simulink model "cop"  (R2020a)
settings: Solver=FixedStepAuto  StartTime=0.0  StopTime=300  FixedStep=1  RelTol=1e-3
undefined symbols (not defined in the file or in its folder): inf_depth, Kc_ini, PGravel
libraries: simulink x4
(part 1 of 2)
settings Model: Creator=KevinChan  LastModifiedBy=KevinChan

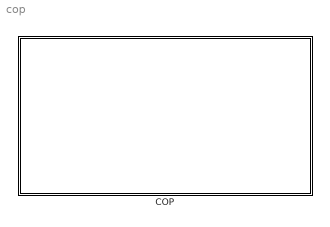
== system cop ==
  COP : Subsystem

== system cop/COP ==
  Climate Model : Subsystem
  Display : Display
  Economic Model : Subsystem
  Gain : Gain  Gain=0.001
  Gain1 : Gain  Gain=0.001
  Integrator : Integrator
  Optimal Irrigation Calculation : Subsystem
  Plant Model : Subsystem
  Scope : Scope  NumInputPorts=2
  Scope1 : Scope
  Soil Model : Subsystem
  Subtract : Sum  Inputs=++-
  VWC : Delay  DelayLength=1  InitialConditionSource=Input port  InitialCondition=0
      settings: InputPortMap=u0,p4
  initial vwc : Constant  Value=0.3
  tag scope: I=global, VWC=global
  wires:
  initial vwc/1 -> VWC/2
  Subtract/1 -> VWC/1, [VWC]
  VWC/1 -> Scope1/1, Subtract/1
  [I] -> Scope/1, Gain1/1
  [WL] -> Scope/2, Gain/1
  Gain/1 -> Subtract/3
  Gain1/1 -> Subtract/2
  Optimal Irrigation Calculation/1(Out1) -> Integrator/1, [I]
  Integrator/1 -> Display/1

== system cop/COP/Climate Model ==
  " Final Calculation for Data" : Subsystem
  " Historic Data" : Subsystem
  AI Forecast Prediction : Subsystem
  General Climate Database : Subsystem  mask{lcation=Palo Alto, Parameter7=No, LatDeg=37, LatMin=28, Altitude=9.1, WindH=2}
      mask prompts: lcation "Select Location"; Parameter7 "More specific Latitude?"; LatDeg "Latitude Degree"; LatMin "Latitude Minute"; Altitude "Altitude above Sea Level [m]"; WindH "Height of measurement above ground surface [m]"
      mask TypeOptions lcation: Palo Alto
      mask TypeOptions Parameter7: Yes | No
      mask DialogControl ParameterGroupVar Prompt: Location
      mask DialogControl Container4 Prompt: If yes, please fill out the following:
      mask DialogControl Container3 Prompt: Wind Measurement (Enter 2 if it uses COP AI Prediction)

== system cop/COP/Economic Model ==

== system cop/COP/Optimal Irrigation Calculation ==
  Constant : Constant  Value=0
  Constant1 : Constant  Value=0
  Display : Display
  Gain : Gain  Gain=0.001
  Gain1 : Gain  Gain=1000
  Math Function : Math  Operator=mod  SaturateOnIntegerOverflow=on
  MinMax : MinMax  Function=max  Inputs=2
  Subtract : Sum  Inputs=++-+
  Switch : Switch  Criteria=u2 ~= 0
  Water Runoff Adjustment : Constant  Value=0
  Out1 : Outport
  wires:
  [qFC] -> Display/1, Subtract/1
  [WL] -> Gain/1
  MinMax/1 -> Gain1/1
  Constant/1 -> MinMax/2
  [VWC] -> Subtract/3
  Subtract/1 -> MinMax/1
  Water Runoff Adjustment/1 -> Subtract/4
  Gain/1 -> Subtract/2
  [DafterPD] -> Math Function/1
  [interval_irr] -> Math Function/2
  Math Function/1 -> Switch/2
  Switch/1 -> Out1/1
  Gain1/1 -> Switch/3
  Constant1/1 -> Switch/1

== system cop/COP/Plant Model ==
  General Plant Database : Subsystem  mask{CropType=Maize (Sweet Corn), PD_Year=2021, PD_Month=2, PD_Day=28, interval_irr_choice=7 days, Parameter18=No, Lini=20, Ldev=40, Lmid=70, Llate=10, Kc_choice=Dual Crop Coefficient, Kc_mid=1.15, Kc_end=1.05, MaxCropH=1.5, Kcb_ini=0.15, Kcb_mid=1.10, Kcb_end=1.00, Zr=1.0}
      mask prompts: CropType "Crop Type"; PD_Year "Year"; PD_Month "Month"; PD_Day "Day"; interval_irr_choice "Interval of Irrigation (0 if unkwon)"; Parameter18 "More specific inputs?"; Lini "Initial Stage"; Ldev "Devloping Stage"; Lmid "Mid-season Stage"; Llate "Late Season Stage"; Kc_choice "Single or Dual Crop Coefficients"; Kc_mid "Enter Kc mid from the Table"; Kc_end "Enter Kc end from the Table"; MaxCropH "Enter Maximum Crop Height (h) (m) from the Table"; Kcb_ini "Enter Kcb ini from the Table"; Kcb_mid "Enter Kcb mid from the Table"; Kcb_end "Enter Kcb end from the Table"; Zr "Enter Zr from the Table"
      mask init:
      | interval_irr = 1;
      | if interval_irr_choice == 1
      |     interval_irr = 1;
      | elseif interval_irr_choice == 2
      |     interval_irr = 2;
      | elseif interval_irr_choice == 3
      |     interval_irr = 4;
      | elseif interval_irr_choice == 4
      |     interval_irr = 7;
      | elseif interval_irr_choice == 5
      |     interval_irr = 10;
      | elseif interval_irr_choice == 6
      |     interval_irr = 20;
      | end
      mask TypeOptions CropType: Maize (Sweet Corn)
      mask TypeOptions interval_irr_choice: 1 day | 2 days | 4 days | 7 days | 10 days | 20 days
      mask TypeOptions Parameter18: Yes | No
      mask TypeOptions Kc_choice: Single Crop Coefficient | Dual Crop Coefficient
      mask DialogControl ParameterGroupVar Prompt: General
      mask DialogControl Control2 Prompt: Plant Date:
      mask DialogControl Control12 Prompt: If yes, please fill out the following:
      mask DialogControl Container3 Prompt: Lengths of Crop Develop Stages
      mask DialogControl Control3 Prompt: Find the values in the following link with corresponding crop type and closest plant date:
      mask DialogControl Control4 Prompt: http://www.fao.org/3/x0490e/x0490e0b.htm#length%20of%20growth%20stages
      mask DialogControl Container4 Prompt: Single Crop Coefficients
      mask DialogControl Control5 Prompt: Find the values for your corresponding crop in the following table:
      mask DialogControl Control6 Prompt: http://www.fao.org/3/x0490e/x0490e0b.htm#tabulated%20kc%20values
      mask DialogControl Container5 Prompt: Dual Crop Coefficents
      mask DialogControl Control7 Prompt: Find the values for your corresponding crop in the following table:
      mask DialogControl Control8 Prompt: http://www.fao.org/3/x0490e/x0490e0c.htm#basal%20crop%20coefficient%20(kcb)
      mask DialogControl Container6 Prompt: Effective Rooting Depth
      mask DialogControl Control10 Prompt: Find the values for your corresponding crop in the following table:
      mask DialogControl Control9 Prompt: http://www.fao.org/3/x0490e/x0490e0e.htm#soil%20water%20availability
  Plant Data Calculation : Subsystem

== system cop/COP/Soil Model ==
  Add : Sum
  Constant : Constant
  Crop Evapotranspiration (ETc) [mm/day] : Product
  Display : Display
  Dual Crop Coefficient (Kcb + Ke) : Subsystem
  Evaporation (ETe) [mm/day] : Product
  General Soil Database : Subsystem  mask{PSand=0.489, PClay=0.170, PSilt=0.341, POM=0.05, fw_choice=Precipitation (fw = 1.0), fw_measured=1, SM_choice=Estimated Soil Moisture Value, qFC_measured=0, qWP_measured=0, Ze_choice=Estimated, Ze_measured=0}
      mask prompts: PSand "Percentage of Sand"; PClay "Percentage of Clay"; PSilt "Percentage of Silt"; POM "Percentage of Organic Matter (0.03-0.06 if unkown)"; fw_choice "Please select the following method (average fw of that method)"; fw_measured "If you selected others or specific fw, please enter your fw value"; SM_choice "Estimated or measured?"; qFC_measured "Field Capacity Soil Moisture (% Volume in m)"; qWP_measured "Wiliting Point Soil Moisture (% Volume in m)"; Ze_choice "Ze estimated or measured?"; Ze_measured "Enter Ze measured if selected"
      mask init:
      | fw = 1
      | if fw_choice == 5
      |     fw = 0.8
      | elseif fw_choice == 6
      |     fw = 0.5
      | elseif fw_choice == 7
      |     fw = 0.4
      | elseif fw_choice == 8
      |     fw = fw_measured
      | end
      mask TypeOptions fw_choice: Precipitation (fw = 1.0) | Sprinkler Irrigation (fw = 1.0) | Basin Irrigation (fw = 1.0) | Border Irrigation (fw = 1.0) | Furrow irrigation (every furrow), narrow bed (fw = 0.6 ... 1.0) | Furrow irrigation (every furrow), wide bed (fw = 0.4 ... 0.6) | Furrow irrigation (alternated furrows) (fw = 0.3 ... 0.5) | Trickle irrigation (fw = 0.3 ... 0.4) | Others or specific fw
      mask TypeOptions SM_choice: Estimated Soil Moisture Value | Measured Soil Moisture Value
      mask TypeOptions Ze_choice: Estimated | Measured
      mask DialogControl ParameterGroupVar Prompt: Percentage of Soil Content (add up to 1)
      mask DialogControl Container7 Prompt: Weight Percentage of Organic Matter
      mask DialogControl Container6 Prompt: Fraction of soil surface wetted by irrigation or precipitation
      mask DialogControl Container3 Prompt: Soil Moisture Data (more accurate if measured)
      mask DialogControl Control3 Prompt: Fill the following if you selected measured
      mask DialogControl Container8 Prompt: Ze depth of the surface soil layer that is subject to drying by way of evaporation [0.10-0.15m]
  Index Vector : MultiPortSwitch  Inputs=2
  Product : Product
  Reference Evapotraspiration (ET0) [mm/day] : Subsystem
  Scope1 : Scope
  Single Crop Coefficient (Kc) : Subsystem
  Soil Data Calculation : Subsystem
  tag scope: E=global, ET0=global, WL=global
  wires:
  Reference Evapotraspiration (ET0) [mm/day]/1(ET0) -> Evaporation (ETe) [mm/day]/1, Crop Evapotranspiration (ETc) [mm/day]/1, [ET0], Display/1
  Single Crop Coefficient (Kc)/1(Out1) -> Index Vector/2
  Index Vector/1 -> Crop Evapotranspiration (ETc) [mm/day]/2
  Dual Crop Coefficient (Kcb + Ke)/2(Ke) -> Evaporation (ETe) [mm/day]/2, Add/2
  Add/1 -> Index Vector/3
  Evaporation (ETe) [mm/day]/1 -> [E]
  [Kc_choice] -> Index Vector/1
  Dual Crop Coefficient (Kcb + Ke)/1(Kcb) -> Scope1/1, Add/1
  Product/1 -> [WL]
  Constant/1 -> Product/2
  Crop Evapotranspiration (ETc) [mm/day]/1 -> Product/1

== system cop/COP/Climate Model/ Final Calculation for Data ==
  Atmospheric Pressure [kPa] : Subsystem
  Daily Temperature [°C] : Subsystem
  Goto12 : Goto  Commented=on  GotoTag=Tpast  TagVisibility=global
  Goto13 : Goto  Commented=on  GotoTag=Tpast_t  TagVisibility=global
  Humidity : Subsystem
  Net Radiation at the Crop Surface (Rn) [MJ/m^2/day] : Subsystem
  Precipitation [mm/day] : Subsystem
  Wind Speed : Subsystem
  tag scope: AP=global, P=global, RHmax=global, RHmean=global, RHmin=global, Rn=global, Tdew=global, Tdry=global, Tmax=global, Tmean=global, Tmin=global, Twet=global, u2=global
  wires:
  Daily Temperature [°C]/1(Tmax) -> [Tmax]
  Daily Temperature [°C]/2(Tmin) -> [Tmin]
  Daily Temperature [°C]/3(Tmean) -> [Tmean]
  Net Radiation at the Crop Surface (Rn) [MJ/m^2/day]/1(Rn) -> [Rn]
  Wind Speed/1(Out1) -> [u2]
  Atmospheric Pressure [kPa]/1(P) -> [AP]
  Daily Temperature [°C]/4(Tdew) -> [Tdew]
  Daily Temperature [°C]/5(Tdry) -> [Tdry]
  Daily Temperature [°C]/6(Twet) -> [Twet]
  Humidity/1(RHmax) -> [RHmax]
  Humidity/3(RHmean) -> [RHmean]
  Humidity/2(RHmin) -> [RHmin]
  Daily Temperature [°C]/7(Tpast) -> Goto12/1
  Daily Temperature [°C]/8(Tpast_time) -> Goto13/1
  Precipitation [mm/day]/1(P) -> [P]

== system cop/COP/Climate Model/ Historic Data ==
  Humidity : Subsystem
  Precipitation : Subsystem
  Solar Radiation : Subsystem
  Temperature [°C] : Subsystem
  "Wind Speed " : Subsystem

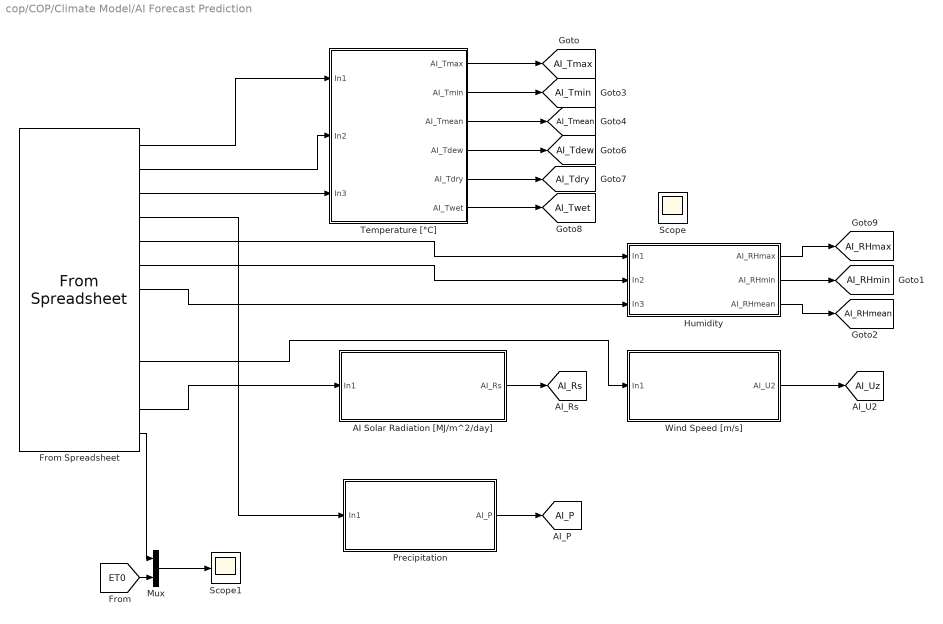
== system cop/COP/Climate Model/AI Forecast Prediction ==
  AI Solar Radiation [MJ/m^2/day] : Subsystem
  From Spreadsheet : FromSpreadsheet  FileName=paloalto3.2020.xlsx  Range=B11:N376  TreatFirstColumnAs=Data  SampleTime=[0,1]
  Humidity : Subsystem
  Mux : Mux  Inputs=2
  Precipitation : Subsystem
  Scope : Scope
  Scope1 : Scope
  Temperature [°C] : Subsystem
  Wind Speed [m/s] : Subsystem
  tag scope: AI_P=global, AI_RHmax=global, AI_RHmean=global, AI_RHmin=global, AI_Rs=global, AI_Tdew=global, AI_Tdry=global, AI_Tmax=global, AI_Tmean=global, AI_Tmin=global, AI_Twet=global, AI_Uz=global
  wires:
  AI Solar Radiation [MJ/m^2/day]/1(AI_Rs) -> [AI_Rs]
  Wind Speed [m/s]/1(AI_U2) -> [AI_Uz]
  Precipitation/1(AI_P) -> [AI_P]
  Humidity/1(AI_RHmax) -> [AI_RHmax]
  Humidity/2(AI_RHmin) -> [AI_RHmin]
  Humidity/3(AI_RHmean) -> [AI_RHmean]
  Temperature [°C]/1(AI_Tmax) -> [AI_Tmax]
  Temperature [°C]/2(AI_Tmin) -> [AI_Tmin]
  Temperature [°C]/3(AI_Tmean) -> [AI_Tmean]
  Temperature [°C]/4(AI_Tdew) -> [AI_Tdew]
  Temperature [°C]/5(AI_Tdry) -> [AI_Tdry]
  Temperature [°C]/6(AI_Twet) -> [AI_Twet]
  [ET0] -> Mux/2
  Mux/1 -> Scope1/1
  From Spreadsheet/1 -> Temperature [°C]/1(In1)
  From Spreadsheet/2 -> Temperature [°C]/2(In2)
  From Spreadsheet/3 -> Temperature [°C]/3(In3)
  From Spreadsheet/13 -> Mux/1
  From Spreadsheet/4 -> Precipitation/1(In1)
  From Spreadsheet/5 -> Humidity/1(In1)
  From Spreadsheet/6 -> Humidity/2(In2)
  From Spreadsheet/7 -> Humidity/3(In3)
  From Spreadsheet/10 -> Wind Speed [m/s]/1(In1)
  From Spreadsheet/12 -> AI Solar Radiation [MJ/m^2/day]/1(In1)

== system cop/COP/Climate Model/General Climate Database ==
  Altitude : Constant  Value=Altitude
  LatDeg : Constant  Value=LatDeg
  LatMin : Constant  Value=LatMin
  WindH : Constant  Value=WindH
  tag scope: Altitude=global, LatDeg=global, LatMin=global, WindH=global
  wires:
  Altitude/1 -> [Altitude]
  LatDeg/1 -> [LatDeg]
  LatMin/1 -> [LatMin]
  WindH/1 -> [WindH]

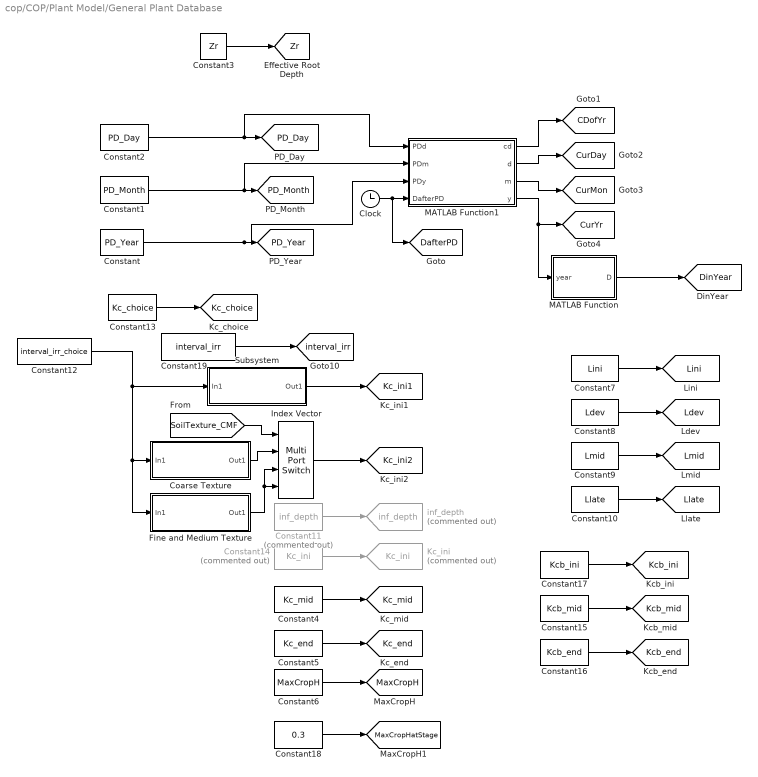
== system cop/COP/Plant Model/General Plant Database ==
  Clock : Clock
  Coarse Texture : Subsystem
  Constant : Constant  Value=PD_Year
  Constant1 : Constant  Value=PD_Month
  Constant10 : Constant  Value=Llate
  Constant11 : Constant  Commented=on  Value=inf_depth
  Constant12 : Constant  Value=interval_irr_choice
  Constant13 : Constant  Value=Kc_choice
  Constant14 : Constant  Commented=on  Value=Kc_ini
  Constant15 : Constant  Value=Kcb_mid
  Constant16 : Constant  Value=Kcb_end
  Constant17 : Constant  Value=Kcb_ini
  Constant18 : Constant  Value=0.3
  Constant19 : Constant  Value=interval_irr
  Constant2 : Constant  Value=PD_Day
  Constant3 : Constant  Value=Zr
  Constant4 : Constant  Value=Kc_mid
  Constant5 : Constant  Value=Kc_end
  Constant6 : Constant  Value=MaxCropH
  Constant7 : Constant  Value=Lini
  Constant8 : Constant  Value=Ldev
  Constant9 : Constant  Value=Lmid
  Fine and Medium Texture : Subsystem
  Index Vector : MultiPortSwitch
  Kc_ini : Goto  Commented=on  GotoTag=Kc_ini  TagVisibility=global
  MATLAB Function : MATLAB Function  TreatAsAtomicUnit=on
  MATLAB Function1 : MATLAB Function  TreatAsAtomicUnit=on
  Subsystem : Subsystem
  inf_depth : Goto  Commented=on  GotoTag=inf_depth  TagVisibility=global
  tag scope: CDofYr=global, CurDay=global, CurMon=global, CurYr=global, DafterPD=global, DinYear=global, Kc_choice=global, Kc_end=global, Kc_ini1=global, Kc_ini2=global, Kc_mid=global, Kcb_end=global, Kcb_ini=global, Kcb_mid=global, Ldev=global, Lini=global, Llate=global, Lmid=global, MaxCropH=global, MaxCropHatStage=global, PD_Day=global, PD_Month=global, PD_Year=global, Zr=global, interval_irr=global
  wires:
  Constant/1 -> MATLAB Function1/3(PDy), [PD_Year]
  Constant1/1 -> MATLAB Function1/2(PDm), [PD_Month]
  Constant2/1 -> MATLAB Function1/1(PDd), [PD_Day]
  MATLAB Function/1(D) -> [DinYear]
  Constant4/1 -> [Kc_mid]
  Constant5/1 -> [Kc_end]
  Constant6/1 -> [MaxCropH]
  Constant9/1 -> [Lmid]
  Constant8/1 -> [Ldev]
  Constant7/1 -> [Lini]
  Constant10/1 -> [Llate]
  Constant11/1 -> inf_depth/1
  [SoilTexture_CMF] -> Index Vector/1
  Index Vector/1 -> [Kc_ini2]
  Constant12/1 -> Subsystem/1(In1), Fine and Medium Texture/1(In1), Coarse Texture/1(In1)
  Subsystem/1(Out1) -> [Kc_ini1]
  Coarse Texture/1(Out1) -> Index Vector/2
  Constant14/1 -> Kc_ini/1
  Clock/1 -> MATLAB Function1/4(DafterPD), [DafterPD]
  MATLAB Function1/1(cd) -> [CDofYr]
  MATLAB Function1/2(d) -> [CurDay]
  MATLAB Function1/3(m) -> [CurMon]
  MATLAB Function1/4(y) -> MATLAB Function/1(year), [CurYr]
  Fine and Medium Texture/1(Out1) -> Index Vector/3, Index Vector/4
  Constant3/1 -> [Zr]
  Constant13/1 -> [Kc_choice]
  Constant16/1 -> [Kcb_end]
  Constant15/1 -> [Kcb_mid]
  Constant17/1 -> [Kcb_ini]
  Constant18/1 -> [MaxCropHatStage]
  Constant19/1 -> [interval_irr]

== system cop/COP/Plant Model/Plant Data Calculation ==
  Constant : Constant  Value=0.05
  MATLAB Function : MATLAB Function  TreatAsAtomicUnit=on
  tag scope: Ph=global, Ps=global
  wires:
  MATLAB Function/1(stage) -> [Ps]
  [DafterPD] -> MATLAB Function/1(d)
  [Lini] -> MATLAB Function/2(Lini)
  [Ldev] -> MATLAB Function/3(Ldev)
  [Lmid] -> MATLAB Function/4(Lmid)
  [Llate] -> MATLAB Function/5(Llate)
  Constant/1 -> [Ph]

== system cop/COP/Soil Model/Dual Crop Coefficient (Kcb + Ke) ==
  Crop Basal Component : Subsystem
  Evaporation Component : Subsystem
  Kcb : Outport
  Ke : Outport  Port=2
  tag scope: Kcb=global
  wires:
  Crop Basal Component/1(Kcb) -> [Kcb], Kcb/1, Evaporation Component/1(Kcb)
  Evaporation Component/1(Ke) -> Ke/1

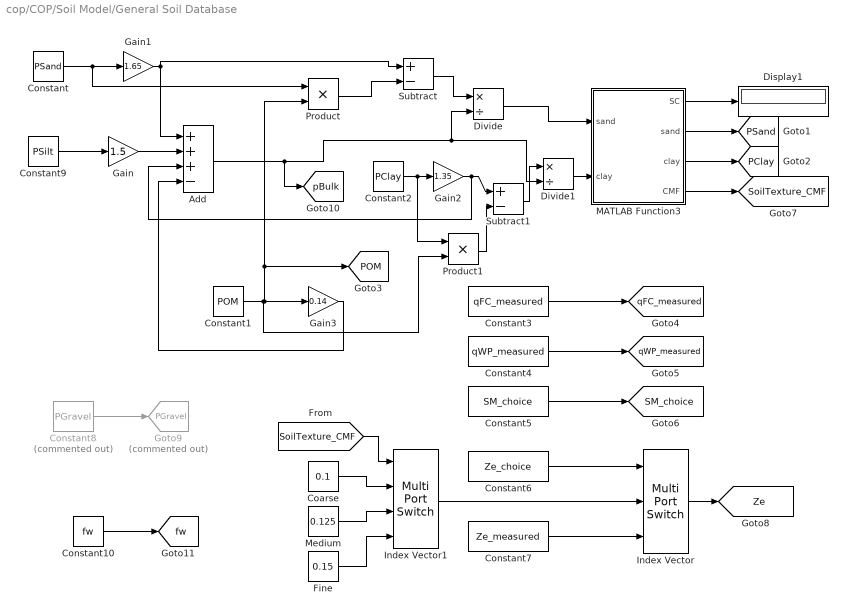
== system cop/COP/Soil Model/General Soil Database ==
  Add : Sum  Inputs=+++-
  Coarse : Constant  Value=0.1
  Constant : Constant  Value=PSand
  Constant1 : Constant  Value=POM
  Constant10 : Constant  Value=fw
  Constant2 : Constant  Value=PClay
  Constant3 : Constant  Value=qFC_measured
  Constant4 : Constant  Value=qWP_measured
  Constant5 : Constant  Value=SM_choice
  Constant6 : Constant  Value=Ze_choice
  Constant7 : Constant  Value=Ze_measured
  Constant8 : Constant  Commented=on  Value=PGravel
  Constant9 : Constant  Value=PSilt
  Display1 : Display
  Divide : Product  Inputs=*/
  Divide1 : Product  Inputs=*/
  Fine : Constant  Value=0.15
  Gain : Gain  Gain=1.5
  Gain1 : Gain  Gain=1.65
  Gain2 : Gain  Gain=1.35
  Gain3 : Gain  Gain=0.14
  Goto9 : Goto  Commented=on  GotoTag=PGravel  TagVisibility=global
  Index Vector : MultiPortSwitch  Inputs=2
  Index Vector1 : MultiPortSwitch
  MATLAB Function3 : MATLAB Function  TreatAsAtomicUnit=on
  Medium : Constant  Value=0.125
  Product : Product
  Product1 : Product
  Subtract : Sum  Inputs=+-
  Subtract1 : Sum  Inputs=+-
  tag scope: PClay=global, POM=global, PSand=global, SM_choice=global, SoilTexture_CMF=global, Ze=global, fw=global, pBulk=global, qFC_measured=global, qWP_measured=global
  wires:
  MATLAB Function3/1(SC) -> Display1/1
  Constant2/1 -> Product1/1, Gain2/1
  Constant/1 -> Product/1, Gain1/1
  Constant3/1 -> [qFC_measured]
  Constant4/1 -> [qWP_measured]
  Constant5/1 -> [SM_choice]
  MATLAB Function3/2(sand) -> [PSand]
  MATLAB Function3/3(clay) -> [PClay]
  MATLAB Function3/4(CMF) -> [SoilTexture_CMF]
  Constant6/1 -> Index Vector/1
  Constant7/1 -> Index Vector/3
  [SoilTexture_CMF] -> Index Vector1/1
  Index Vector1/1 -> Index Vector/2
  Coarse/1 -> Index Vector1/2
  Fine/1 -> Index Vector1/4
  Medium/1 -> Index Vector1/3
  Index Vector/1 -> [Ze]
  Constant8/1 -> Goto9/1
  Constant9/1 -> Gain/1
  Gain1/1 -> Subtract/1, Add/1
  Gain2/1 -> Subtract1/1, Add/3
  Gain/1 -> Add/2
  Gain3/1 -> Add/4
  Add/1 -> Divide1/2, Divide/2, [pBulk]
  Divide/1 -> MATLAB Function3/1("sand ")
  Divide1/1 -> MATLAB Function3/2("clay ")
  Subtract/1 -> Divide/1
  Constant1/1 -> Product1/2, [POM], Product/2, Gain3/1
  Product/1 -> Subtract/2
  Subtract1/1 -> Divide1/1
  Product1/1 -> Subtract1/2
  Constant10/1 -> [fw]

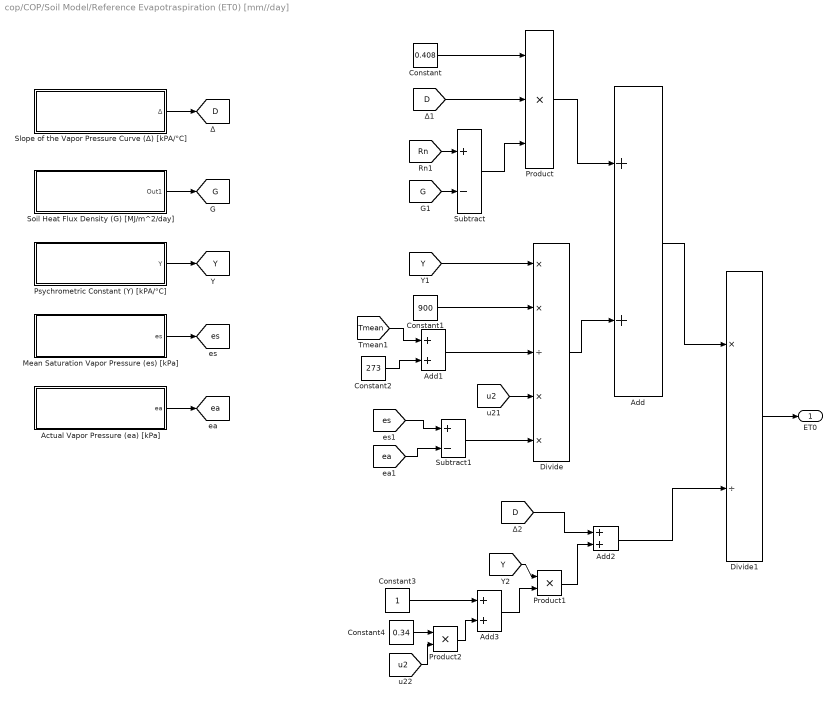
== system cop/COP/Soil Model/Reference Evapotraspiration (ET0) [mm//day] ==
  Actual Vapor Pressure (ea) [kPa] : Subsystem  mask{ea_choice=Derived from Dewpoint Temperature, apsy_choice=0.000662 for ventilated (Asmann type) psychrometers, with an air movement of some 5 m/s}
      mask prompts: ea_choice "Select which method to derive:"; apsy_choice "Pick value for apsy:"
      mask init:
      | apsy = 0;
      | 
      | if apsy_choice == 1
      |     apsy = 0.000662;
      | elseif apsy_choice == 2
      |     apsy = 0.000800;
      | elseif apsy_choice == 3
      |     apsy = 0.001200;
      | end
      mask TypeOptions ea_choice: Derived from Dewpoint Temperature | Derived from Psyschrometirc Data | Derived from Relative Humidity Data (RHmax and RHmin) | Derived from Relative Humidity Data (RHmax only) | Derived from Relative Humidity Data (RHmean only)
      mask TypeOptions apsy_choice: 0.000662 for ventilated (Asmann type) psychrometers, with an air movement of some 5 m/s | 0.000800 for natural ventilated psychrometers (about 1 m/s) | 0.001200 for non-ventilated psychrometers installed indoors.
      mask DialogControl Control2 Prompt: There are 3 different ways to derive the actual vapor pressure. Depend on what data you have avaliable, pick the following choices. If you are picking relatitive humidity, beware of the following. When using equipment where errors in estimating RHmin can be large, or when RH data integrity are in doubt, then one should use only RHmax. In the absence of RHmax and RHmin, you can select to use RHmean.
      mask DialogControl Control3 Prompt: If you picked to use Psychrometric Data, select the folowing.
  Add{,1..3} (4 alike) : Sum
  Constant : Constant  Value=0.408
  Constant1 : Constant  Value=900
  Constant2 : Constant  Value=273
  Constant3 : Constant
  Constant4 : Constant  Value=0.34
  Divide : Product  Inputs=**/**
  Divide1 : Product  Inputs=*/
  "Mean Saturation Vapor Pressure (es) [kPa] " : Subsystem
  Product : Product  Inputs=3
  Product1 : Product
  Product2 : Product
  Psychrometric Constant (Y) [kPA/°C] : Subsystem
  Slope of the Vapor Pressure Curve (∆) [kPA/°C] : Subsystem
  Soil Heat Flux Density (G) [MJ/m^2/day] : Subsystem  mask{G_choice=For long periods}
      mask prompts: G_choice "Select Time Step:"
      mask TypeOptions G_choice: For day and ten-day periods | For long periods
      mask DialogControl Control2 Prompt: For daily or weekly periods of time, soil heat flux density is small and can be ignored. A method to find G for long period of time is here, based on the idea that the soil temperature follows air temperature.
  Subtract : Sum  Inputs=+-
  Subtract1 : Sum  Inputs=+-
  ET0 : Outport
  tag scope: D=global, G=global, Y=global, ea=global, es=global
  wires:
  Divide1/1 -> ET0/1
  Constant/1 -> Product/1
  [D] -> Product/2
  [Rn] -> Subtract/1
  [G] -> Subtract/2
  Subtract/1 -> Product/3
  Product/1 -> Add/1
  Divide/1 -> Add/2
  Constant1/1 -> Divide/2
  [Tmean] -> Add1/1
  Constant2/1 -> Add1/2
  Add1/1 -> Divide/3
  Subtract1/1 -> Divide/5
  [es] -> Subtract1/1
  [ea] -> Subtract1/2
  Add/1 -> Divide1/1
  Add2/1 -> Divide1/2
  Product1/1 -> Add2/2
  Add3/1 -> Product1/2
  Constant3/1 -> Add3/1
  Product2/1 -> Add3/2
  Slope of the Vapor Pressure Curve (∆) [kPA/°C]/1(∆) -> [D]
  [D] -> Add2/1
  Soil Heat Flux Density (G) [MJ/m^2/day]/1(Out1) -> [G]
  Psychrometric Constant (Y) [kPA/°C]/1(Y) -> [Y]
  [Y] -> Divide/1
  [Y] -> Product1/1
  [u2] -> Divide/4
  [u2] -> Product2/2
  "Mean Saturation Vapor Pressure (es) [kPa] "/1(es) -> [es]
  Actual Vapor Pressure (ea) [kPa]/1(ea) -> [ea]
  Constant4/1 -> Product2/1

== system cop/COP/Soil Model/Single Crop Coefficient (Kc) ==
  Adjustment to Crop Coefficient : Subsystem
  Constant : Constant  Value=0
  Development Stage : Subsystem
  Index Vector : MultiPortSwitch  DataPortOrder=Zero-based contiguous  Inputs=5  zeroidx=on
  Initial Stage : Subsystem
  Late Season Stage : Subsystem
  Mid-season Stage : Subsystem
  Switch : Switch  Criteria=u2 > Threshold  Threshold=10
  Switch1 : Switch  Criteria=u2 > Threshold  Threshold=40
  Out1 : Outport
  wires:
  Index Vector/1 -> Out1/1
  [Ps] -> Index Vector/1
  Mid-season Stage/1(Kc mid) -> Late Season Stage/1(Kc mid), Index Vector/4, Development Stage/2(Kc mid)
  Adjustment to Crop Coefficient/1(Kc_adj) -> Late Season Stage/2(Kc_adj), Mid-season Stage/1(Kc_adj)
  Development Stage/1(Out1) -> Index Vector/3
  Late Season Stage/1(Out1) -> Index Vector/5
  Switch/1 -> Index Vector/2, Development Stage/1(Kc ini)
  [Kc_ini1] -> Switch/3
  [interval_irr] -> Switch1/2, Switch/2
  Constant/1 -> Index Vector/6
  Switch1/1 -> Switch/1
  Initial Stage/1(Out1) -> Switch1/3
  [Kc_ini2] -> Switch1/1

== system cop/COP/Soil Model/Soil Data Calculation ==
  Constant : Constant  Value=0
  Constant1 : Constant  Value=0
  Demux : Demux  Outputs=2
  Estimated Soil Heat Capacity (UC Davis) : Subsystem
  Estimated qFC (Saxton and Rawls Function) : Subsystem
  Estimated qWP (Saxton and Rawls Function) : Subsystem
  Index Vector : MultiPortSwitch  Inputs=2
  Mux : Mux  Inputs=2
  Mux1 : Mux  Inputs=2
  tag scope: RO=global, Te=global, cs=global, qFC=global, qWP=global
  wires:
  [SM_choice] -> Index Vector/1
  [qFC_measured] -> Mux/1
  [qWP_measured] -> Mux/2
  Mux/1 -> Index Vector/3
  Index Vector/1 -> Demux/1
  Demux/1 -> [qFC]
  Demux/2 -> [qWP]
  Mux1/1 -> Index Vector/2
  Estimated qFC (Saxton and Rawls Function)/1(" θ33 or qFC") -> Mux1/1
  Estimated qWP (Saxton and Rawls Function)/1(θ1500 or qWP) -> Mux1/2
  Estimated Soil Heat Capacity (UC Davis)/1(Out1) -> [cs]
  Constant/1 -> [RO]
  Constant1/1 -> [Te]

== system cop/COP/Climate Model/ Final Calculation for Data/Atmospheric Pressure [kPa] ==
  Constant : Constant  Value=101.3
  Constant1 : Constant  Value=5.26
  Constant2 : Constant  Value=293
  Constant3 : Constant  Value=0.0065
  Constant5 : Constant  Value=293
  Divide : Product  Inputs=*/
  Math Function : Math  Operator=pow  SaturateOnIntegerOverflow=on
  Product : Product
  Product1 : Product
  Subtract : Sum  Inputs=+-
  P : Outport
  wires:
  Product/1 -> P/1
  Constant/1 -> Product/1
  Math Function/1 -> Product/2
  Constant1/1 -> Math Function/2
  Divide/1 -> Math Function/1
  Subtract/1 -> Divide/1
  Constant2/1 -> Subtract/1
  Product1/1 -> Subtract/2
  Constant3/1 -> Product1/1
  [Altitude] -> Product1/2
  Constant5/1 -> Divide/2

== system cop/COP/Climate Model/ Final Calculation for Data/Daily Temperature [°C] ==
  Display : Display
  Humidity Formula for Dew Point : Subsystem
  Manual Switch : ManualSwitch
  Mean Air Temperature at 2m height (Tmean) [°C] : Subsystem
  Tmax : Outport
  Tmin : Outport  Port=2
  Tmean : Outport  Port=3
  Tdew : Outport  Port=4
  Tdry : Outport  Port=5
  Twet : Outport  Port=6
  Tpast : Outport  Port=7
  Tpast_time : Outport  Port=8
  wires:
  [AI_Tmax] -> Tmax/1
  [AI_Tmin] -> Tmin/1
  [AI_Tmean] -> Tmean/1
  [AI_Tdry] -> Tdry/1
  [AI_Twet] -> Twet/1
  [AI_Tdew] -> Manual Switch/2
  Manual Switch/1 -> Display/1, Tdew/1
  Humidity Formula for Dew Point/1(Out1) -> Manual Switch/1

== system cop/COP/Climate Model/ Final Calculation for Data/Humidity ==
  RHmax : Outport
  RHmin : Outport  Port=2
  RHmean : Outport  Port=3
  wires:
  [AI_RHmax] -> RHmax/1
  [AI_RHmin] -> RHmin/1
  [AI_RHmean] -> RHmean/1

== system cop/COP/Climate Model/ Final Calculation for Data/Net Radiation at the Crop Surface (Rn) [MJ//m^2//day] ==
  Clear-Sky Solar Radiation (Rso) [MJ/m^2/day] : Subsystem
  Extraterrestrial Radiation (Ra) [MJ/m^2/day] : Subsystem
  Net Longwave Radiation (Rnl) [MJ/m^2/day] : Subsystem
  Net Solar/Shortwave Radiation (Rns) [MJ/m^2/day] : Subsystem
  Solar Radiation (Rs) [MJ/m^2/day] : Subsystem  mask{Ac_Rs=AI Predicted Solar Radiation}
      mask prompts: Ac_Rs "How to calculate Solar Radiation? (Most to Least Accurate)"
      mask TypeOptions Ac_Rs: AI Predicted Solar Radiation | Angstrom Formula if AI_Rs not avaliable | Hargreaves Formula if AI_Rs and hour of daylight is not available
  Subtract : Sum  Inputs=+-
  Rn : Outport
  tag scope: Ra=global, Rs=global, Rso=global
  wires:
  Subtract/1 -> Rn/1
  Net Solar/Shortwave Radiation (Rns) [MJ/m^2/day]/1(Out1) -> Subtract/1
  Net Longwave Radiation (Rnl) [MJ/m^2/day]/1(Rnl) -> Subtract/2
  Solar Radiation (Rs) [MJ/m^2/day]/1(Rs) -> [Rs]
  Extraterrestrial Radiation (Ra) [MJ/m^2/day]/1(Ra) -> [Ra]
  [CDofYr] -> Extraterrestrial Radiation (Ra) [MJ/m^2/day]/1(J)
  Clear-Sky Solar Radiation (Rso) [MJ/m^2/day]/1(Rso) -> [Rso]

== system cop/COP/Climate Model/ Final Calculation for Data/Precipitation [mm//day] ==
  P : Outport
  wires:
  [AI_P] -> P/1

== system cop/COP/Climate Model/ Final Calculation for Data/Wind Speed ==
  Wind Speed measured at 2m height (u2) [m/s] : Subsystem
  Out1 : Outport
  wires:
  Wind Speed measured at 2m height (u2) [m/s]/1(u2) -> Out1/1
  [WindH] -> Wind Speed measured at 2m height (u2) [m/s]/2(z)
  [AI_Uz] -> Wind Speed measured at 2m height (u2) [m/s]/1(uz)

== system cop/COP/Climate Model/ Historic Data/Humidity ==

== system cop/COP/Climate Model/ Historic Data/Precipitation ==

== system cop/COP/Climate Model/ Historic Data/Solar Radiation ==

== system cop/COP/Climate Model/ Historic Data/Temperature [°C] ==

== system cop/COP/Climate Model/ Historic Data/Wind Speed  ==

== system cop/COP/Climate Model/AI Forecast Prediction/AI Solar Radiation [MJ//m^2//day] ==
  In1 : Inport
  AI_Rs : Outport
  wires:
  In1/1 -> AI_Rs/1

== system cop/COP/Climate Model/AI Forecast Prediction/Humidity ==
  In1 : Inport
  In2 : Inport  Port=2
  In3 : Inport  Port=3
  AI_RHmax : Outport
  AI_RHmin : Outport  Port=2
  AI_RHmean : Outport  Port=3
  wires:
  In1/1 -> AI_RHmax/1
  In2/1 -> AI_RHmin/1
  In3/1 -> AI_RHmean/1

== system cop/COP/Climate Model/AI Forecast Prediction/Precipitation ==
  In1 : Inport
  AI_P : Outport
  wires:
  In1/1 -> AI_P/1

== system cop/COP/Climate Model/AI Forecast Prediction/Temperature [°C] ==
  In1 : Inport
  In2 : Inport  Port=2
  In3 : Inport  Port=3
  AI_Tmax : Outport
  AI_Tmin : Outport  Port=2
  AI_Tmean : Outport  Port=3
  AI_Tdew : Outport  Port=4
  AI_Tdry : Outport  Port=5
  AI_Twet : Outport  Port=6
  wires:
  In1/1 -> AI_Tmax/1
  In2/1 -> AI_Tmin/1
  In3/1 -> AI_Tmean/1

== system cop/COP/Climate Model/AI Forecast Prediction/Wind Speed [m//s] ==
  In1 : Inport
  AI_U2 : Outport
  wires:
  In1/1 -> AI_U2/1

== system cop/COP/Plant Model/General Plant Database/Coarse Texture ==
  In1 : Inport
  2-D Lookup Table : Lookup_n-D  BreakpointsForDimension1=[0 1 2 3 4 5 6 7 8 9 10 11 12]  BreakpointsForDimension2=[1 2 3 4 5 6]  Table=|  InternalRulePriority=Speed  RndMeth=Simplest  InputSameDT=on
      | [1.15 1.15 1.15 1.15 1.15 1.15;
      | 1.15 1.15 1.15 1 0.7 0.35;
      | 1.15 1.15 1.05 0.7 0.5 0.25;
      | 1.15 1.15 0.875 0.575 0.4 0.2;
      | 1.15 1.075 0.775 0.425 0.35 0.175;
      | 1.15 1 0.65 0.4 0.28 0.15;
      | 1.13 0.94 0.575 0.35 0.25 0.125;
      | 1.1 0.86 0.52 0.3 0.21 0.1;
      | 1.075 0.8 0.45 0.27 0.18 0.08;
      | 1.05 0.73 0.41 0.23 0.16 0.07;
      | 1.01 0.675 0.375 0.21 0.14 0.06;
      | 0.975 0.63 0.34 0.19 0.13 0.055;
      | 0.925 0.6 0.31 0.175 0.12 0.05]
  Round : Rounding  Operator=round
  Out1 : Outport
  wires:
  [ET0] -> Round/1
  2-D Lookup Table/1 -> Out1/1
  In1/1 -> 2-D Lookup Table/2
  Round/1 -> 2-D Lookup Table/1

== system cop/COP/Plant Model/General Plant Database/Fine and Medium Texture ==
  In1 : Inport
  2-D Lookup Table : Lookup_n-D  BreakpointsForDimension1=[0 1 2 3 4 5 6 7 8 9 10 11 12]  BreakpointsForDimension2=[1 2 3 4 5 6]  Table=|  InternalRulePriority=Speed  RndMeth=Simplest  InputSameDT=on
      | [1.15 1.15 1.15 1.15 1.15 1.15;
      | 1.15 1.15 1.15 1.15 1.15 0.65;
      | 1.15 1.15 1.15 1.125 0.85 0.45;
      | 1.15 1.15 1.1 0.87 0.7 0.38;
      | 1.15 1.15 1.025 0.7 0.6 0.325;
      | 1.15 1.125 0.95 0.65 0.5 0.275;
      | 1.15 1.1 0.875 0.6 0.45 0.225;
      | 1.15 1.06 0.81 0.54 0.4 0.2;
      | 1.15 1.025 0.73 0.48 0.35 0.175;
      | 1.14 0.98 0.675 0.43 0.3 0.15;
      | 1.125 0.94 0.63 0.39 0.275 0.125;
      | 1.1 0.9 0.59 0.35 0.25 0.11;
      | 1.08 0.85 0.55 0.31 0.225 0.1]
  Round : Rounding  Operator=round
  Out1 : Outport
  wires:
  2-D Lookup Table/1 -> Out1/1
  [ET0] -> Round/1
  In1/1 -> 2-D Lookup Table/2
  Round/1 -> 2-D Lookup Table/1

== system cop/COP/Plant Model/General Plant Database/Subsystem ==
  In1 : Inport
  2-D Lookup Table : Lookup_n-D  BreakpointsForDimension1=[0 1 2 3 4 5 6 7 8 9 10 11 12]  BreakpointsForDimension2=[1 2 3 4 5 6]  Table=|  InternalRulePriority=Speed  RndMeth=Simplest  InputSameDT=on
      | [1.15 1.15 1.15 1.15 1.15 1.15; 
      | 1.15 1.15 1.15 1.15 0.9 0.5; 
      | 1.15 1.15 1 0.675 0.5 0.25;
      | 1.15 1.05 0.7 0.475 0.325 0.175;
      | 1.1 0.9 0.6 0.35 0.25 0.125;
      | 1.05 0.775 0.475 0.275 0.2 0.1;
      | 0.95 0.7 0.41 0.225 0.175 0.08;
      | 0.9 0.625 0.35 0.21 0.15 0.07;
      | 0.875 0.575 0.3 0.18 0.125 0.06;
      | 0.825 0.525 0.275 0.16 0.11 0.05;
      | 0.775 0.475 0.25 0.14 0.1 0.045;
      | 0.725 0.425 0.225 0.125 0.09 0.04;
      | 0.7 0.4 0.2 0.11 0.08 0.04]
  Round : Rounding  Operator=round
  Out1 : Outport
  wires:
  In1/1 -> 2-D Lookup Table/2
  2-D Lookup Table/1 -> Out1/1
  [ET0] -> Round/1
  Round/1 -> 2-D Lookup Table/1

== system cop/COP/Soil Model/Dual Crop Coefficient (Kcb + Ke)/Crop Basal Component ==
  Adjustment to Crop Coefficient : Subsystem
  Constant : Constant  Value=0
  Development Stage : Subsystem
  Index Vector : MultiPortSwitch  DataPortOrder=Zero-based contiguous  Inputs=5  zeroidx=on
  Late Season Stage : Subsystem
  Mid-season Stage : Subsystem
  Kcb : Outport
  wires:
  Index Vector/1 -> Kcb/1
  [Ps] -> Index Vector/1
  Development Stage/1(Out1) -> Index Vector/3
  Late Season Stage/1(Out1) -> Index Vector/5
  Mid-season Stage/1(Kcb mid) -> Development Stage/2(Kcb mid), Index Vector/4, Late Season Stage/1(Kcb mid)
  Adjustment to Crop Coefficient/1(Kcb_adj) -> Late Season Stage/2(Kcb_adj), Mid-season Stage/1(Kcb_adj)
  [Kcb_ini] -> Development Stage/1(Kcb ini), Index Vector/2
  Constant/1 -> Index Vector/6

== system cop/COP/Soil Model/Dual Crop Coefficient (Kcb + Ke)/Evaporation Component ==
  Kcb : Inport
  Constant : Constant
  Exposed and wetted soil fraction (few) : Subsystem
  Index Vector : MultiPortSwitch  DataPortOrder=Zero-based contiguous  Inputs=2  zeroidx=on
  MinMax : MinMax  Inputs=2
  Product : Product
  Product1 : Product
  Relational Operator : RelationalOperator  Operator=>  OutDataTypeStr=boolean  RndMeth=Simplest
  Soil evaporation reduction coefficient (Kr) : Subsystem
  Subtract : Sum  Inputs=+-
  Upper Limit (Kc max) : Subsystem
  Ke : Outport
  tag scope: Kc_max=global, few=global
  wires:
  Kcb/1 -> Upper Limit (Kc max)/1(Kcb), Subtract/2
  Upper Limit (Kc max)/1(Out1) -> [Kc_max], Subtract/1, Product1/2
  Subtract/1 -> Product/2
  Product/1 -> MinMax/1
  MinMax/1 -> Ke/1
  [De_past] -> Relational Operator/1
  Relational Operator/1 -> Index Vector/1
  [REW] -> Relational Operator/2
  Constant/1 -> Index Vector/2
  Soil evaporation reduction coefficient (Kr)/1(Out1) -> Index Vector/3
  Index Vector/1 -> Product/1
  Product1/1 -> MinMax/2
  Exposed and wetted soil fraction (few)/1(Out1) -> Product1/1, [few]

== system cop/COP/Soil Model/Reference Evapotraspiration (ET0) [mm//day]/Actual Vapor Pressure (ea) [kPa] ==
  Constant : Constant  Value=ea_choice
  Derived from Dewpoint Temperature : Subsystem
  Derived from Psychrometric Data : Subsystem
  Derived from RHmax & RHmin : Subsystem
  Derived from RHmax only : Subsystem
  Derived from RHmean only : Subsystem
  Index Vector : MultiPortSwitch  Inputs=5
  ea : Outport
  wires:
  Derived from Dewpoint Temperature/1(Out1) -> Index Vector/2
  Index Vector/1 -> ea/1
  Constant/1 -> Index Vector/1
  Derived from Psychrometric Data/1(Out1) -> Index Vector/3
  Derived from RHmean only/1(Out1) -> Index Vector/6
  Derived from RHmax only/1(Out1) -> Index Vector/5
  Derived from RHmax & RHmin/1(Out1) -> Index Vector/4

== system cop/COP/Soil Model/Reference Evapotraspiration (ET0) [mm//day]/Mean Saturation Vapor Pressure (es) [kPa]  ==
  Add2 : Sum
  Constant6 : Constant  Value=2
  Divide2 : Product  Inputs=*/
  Saturation Vapor Pressure (eo) : Subsystem
  Saturation Vapor Pressure (eo) 2 : Subsystem
  es : Outport
  wires:
  Add2/1 -> Divide2/1
  Divide2/1 -> es/1
  Constant6/1 -> Divide2/2
  [Tmax] -> Saturation Vapor Pressure (eo)/1(In1)
  Saturation Vapor Pressure (eo)/1(Out1) -> Add2/1
  [Tmin] -> Saturation Vapor Pressure (eo) 2/1(In1)
  Saturation Vapor Pressure (eo) 2/1(Out1) -> Add2/2

== system cop/COP/Soil Model/Reference Evapotraspiration (ET0) [mm//day]/Psychrometric Constant (Y) [kPA//°C] ==
  Divide : Product  Inputs=**//
  Latent Heat of Vaporization (l) [MJ/kg] : Subsystem
  Ratio Molecular Weight of Water Vapour/Dry Air (e) : Constant  Value=0.622
  "Specific Heat at Constant Pressure (cp) [MJ/kg/°C] " : Constant  Value=0.001013
  Y : Outport
  wires:
  Divide/1 -> Y/1
  "Specific Heat at Constant Pressure (cp) [MJ/kg/°C] "/1 -> Divide/1
  Latent Heat of Vaporization (l) [MJ/kg]/1(l) -> Divide/4
  [AP] -> Divide/2
  Ratio Molecular Weight of Water Vapour/Dry Air (e)/1 -> Divide/3

== system cop/COP/Soil Model/Reference Evapotraspiration (ET0) [mm//day]/Slope of the Vapor Pressure Curve (∆) [kPA//°C] ==
  Add : Sum
  Constant : Constant  Value=4098
  Constant1 : Constant  Value=0.6108
  Constant2 : Constant  Value=17.27
  Constant3 : Constant  Value=237.3
  Divide : Product  Inputs=***//
  Divide1 : Product  Inputs=**/
  Math Function : Math  SaturateOnIntegerOverflow=on
  ∆ : Outport
  wires:
  Divide/1 -> ∆/1
  Constant/1 -> Divide/1
  Constant1/1 -> Divide/2
  Math Function/1 -> Divide/3
  Divide1/1 -> Math Function/1
  [Tmean] -> Add/1, Divide1/2
  Constant2/1 -> Divide1/1
  Add/1 -> Divide/5, Divide/4, Divide1/3
  Constant3/1 -> Add/2

== system cop/COP/Soil Model/Reference Evapotraspiration (ET0) [mm//day]/Soil Heat Flux Density (G) [MJ//m^2//day] ==
  note: Since the model is modeling each day of the year, so it is a daily period
  Constant : Constant  Commented=on  Value=G_choice
  For day and ten-day peroids : Constant  Value=0
  Index Vector : MultiPortSwitch  Commented=on  Inputs=2
  Long Time Steps : Subsystem  Commented=on
  Out1 : Outport
  wires:
  Long Time Steps/1(Out1) -> Index Vector/3
  For day and ten-day peroids/1 -> Out1/1
  Constant/1 -> Index Vector/1

== system cop/COP/Soil Model/Single Crop Coefficient (Kc)/Adjustment to Crop Coefficient ==
  Constant2 : Constant  Value=0.3
  Constant3 : Constant  Value=3
  Constant4 : Constant  Value=0.004
  Constant5 : Constant  Value=45
  Constant6 : Constant  Value=0.04
  Constant7 : Constant  Value=2
  Divide : Product  Inputs=*/
  Math Function : Math  Operator=pow  SaturateOnIntegerOverflow=on
  Product : Product
  Product1 : Product
  Product2 : Product
  Subtract : Sum  Inputs=+-
  Subtract1 : Sum  Inputs=+-
  Subtract2 : Sum  Inputs=+-
  Kc_adj : Outport
  wires:
  Product/1 -> Kc_adj/1
  Subtract/1 -> Product/1
  [u2] -> Subtract2/1
  Constant4/1 -> Product1/1
  Constant7/1 -> Subtract2/2
  [RHmin] -> Subtract1/1
  Product1/1 -> Subtract/2
  Constant5/1 -> Subtract1/2
  Divide/1 -> Math Function/1
  Constant3/1 -> Divide/2
  Constant2/1 -> Math Function/2
  Product2/1 -> Subtract/1
  [MaxCropHatStage] -> Divide/1
  Subtract2/1 -> Product2/2
  Math Function/1 -> Product/2
  Subtract1/1 -> Product1/2
  Constant6/1 -> Product2/1

== system cop/COP/Soil Model/Single Crop Coefficient (Kc)/Development Stage ==
  Kc ini : Inport
  Kc mid : Inport  Port=2
  Add : Sum
  Divide : Product  Inputs=*/
  Product : Product
  Subtract : Sum  Inputs=+-
  Subtract1 : Sum  Inputs=+-
  Out1 : Outport
  wires:
  Add/1 -> Out1/1
  Kc ini/1 -> Add/1, Subtract/2
  Product/1 -> Add/2
  Subtract/1 -> Product/2
  Kc mid/1 -> Subtract/1
  Divide/1 -> Product/1
  [Ldev] -> Divide/2
  Subtract1/1 -> Divide/1
  [Lini] -> Subtract1/2
  [DafterPD] -> Subtract1/1

== system cop/COP/Soil Model/Single Crop Coefficient (Kc)/Initial Stage ==
  Add : Sum
  Constant2 : Constant  Value=10
  Constant3 : Constant  Value=40
  Constant4 : Constant  Value=10
  Divide : Product  Inputs=*/*
  Subtract : Sum  Inputs=+-
  Subtract1 : Sum  Inputs=+-
  Subtract2 : Sum  Inputs=+-
  Out1 : Outport
  wires:
  Add/1 -> Out1/1
  [Kc_ini1] -> Add/1, Subtract2/2
  Divide/1 -> Add/2
  Subtract/1 -> Divide/1
  [I] -> Subtract/1
  Constant2/1 -> Subtract/2
  Subtract1/1 -> Divide/2
  Constant3/1 -> Subtract1/1
  Constant4/1 -> Subtract1/2
  Subtract2/1 -> Divide/3
  [Kc_ini2] -> Subtract2/1

== system cop/COP/Soil Model/Single Crop Coefficient (Kc)/Late Season Stage ==
  Kc mid : Inport
  Kc_adj : Inport  Port=2
  Add : Sum
  Add1 : Sum
  Add2 : Sum  Inputs=+++
  Divide : Product  Inputs=*/
  Product : Product
  Subtract : Sum  Inputs=+-
  Subtract1 : Sum  Inputs=+-
  Out1 : Outport
  wires:
  [Kc_end] -> Add/1
  Kc_adj/1 -> Add/2
  Subtract/1 -> Product/2
  Divide/1 -> Product/1
  [DafterPD] -> Subtract1/1
  Add1/1 -> Out1/1
  Product/1 -> Add1/2
  [Llate] -> Divide/2
  Kc mid/1 -> Add1/1, Subtract/2
  Subtract1/1 -> Divide/1
  Add/1 -> Subtract/1
  Add2/1 -> Subtract1/2
  [Lini] -> Add2/1
  [Ldev] -> Add2/2
  [Lmid] -> Add2/3

== system cop/COP/Soil Model/Single Crop Coefficient (Kc)/Mid-season Stage ==
  Kc_adj : Inport
  Add : Sum
  Kc mid : Outport
  wires:
  Add/1 -> Kc mid/1
  Kc_adj/1 -> Add/2
  [Kc_mid] -> Add/1

== system cop/COP/Soil Model/Soil Data Calculation/Estimated Soil Heat Capacity (UC Davis) ==
  Add : Sum
  Bulk Density (Saxton and Rawls Function) [g/cm^3) : Subsystem  Commented=on
  Constant : Constant  Value=837
  Constant1 : Constant  Value=4.19*10^6
  Gain : Gain  Gain=0.001
  Product : Product
  Product1 : Product
  Out1 : Outport
  wires:
  Add/1 -> Out1/1
  Constant/1 -> Product/1
  Product/1 -> Add/1
  Product1/1 -> Add/2
  Constant1/1 -> Product1/1
  [VWC] -> Product1/2
  Gain/1 -> Product/2
  [pBulk] -> Gain/1

== system cop/COP/Soil Model/Soil Data Calculation/Estimated qFC (Saxton and Rawls Function) ==
  Constant : Constant  Value=1.283
  Constant1 : Constant  Value=0.015
  Constant2 : Constant  Value=0.374
  Product : Product  Inputs=3
  Product1 : Product
  Subtract : Sum  Inputs=++--
  θ33t : Subsystem
  " θ33 or qFC" : Outport
  wires:
  θ33t/1(Out1) -> Product1/1, Product/2, Product/1, Subtract/1
  Product/1 -> Subtract/2
  Constant/1 -> Product/3
  Constant1/1 -> Subtract/4
  Subtract/1 -> " θ33 or qFC"/1
  Product1/1 -> Subtract/3
  Constant2/1 -> Product1/2

== system cop/COP/Soil Model/Soil Data Calculation/Estimated qWP (Saxton and Rawls Function) ==
  Constant : Constant  Value=0.14
  Constant1 : Constant  Value=0.02
  Product : Product
  Subtract : Sum  Inputs=++-
  θ1500t : Subsystem
  θ1500 or qWP : Outport
  wires:
  Subtract/1 -> θ1500 or qWP/1
  Constant/1 -> Product/2
  θ1500t/1(Out1) -> Subtract/1, Product/1
  Constant1/1 -> Subtract/3
  Product/1 -> Subtract/2

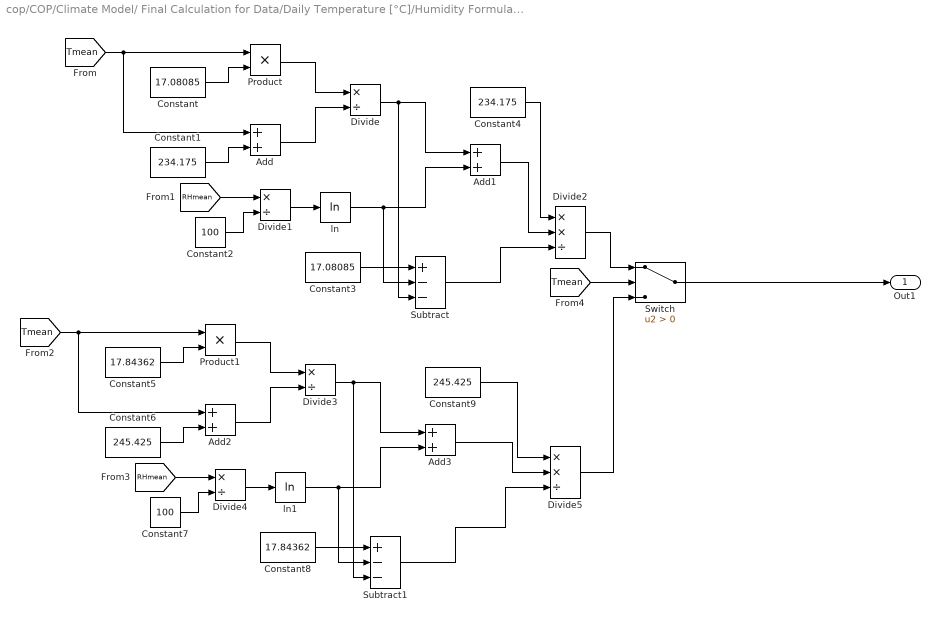
== system cop/COP/Climate Model/ Final Calculation for Data/Daily Temperature [°C]/Humidity Formula for Dew Point ==
  Add{,1..3} (4 alike) : Sum
  Constant : Constant  Value=17.08085
  Constant1 : Constant  Value=234.175
  Constant2 : Constant  Value=100
  Constant3 : Constant  Value=17.08085
  Constant4 : Constant  Value=234.175
  Constant5 : Constant  Value=17.84362
  Constant6 : Constant  Value=245.425
  Constant7 : Constant  Value=100
  Constant8 : Constant  Value=17.84362
  Constant9 : Constant  Value=245.425
  Divide{,1,3..4} (4 alike) : Product  Inputs=*/
  Divide2 : Product  Inputs=**/
  Divide5 : Product  Inputs=**/
  Product : Product
  Product1 : Product
  Subtract : Sum  Inputs=+--
  Subtract1 : Sum  Inputs=+--
  Switch : Switch  Criteria=u2 > Threshold
  ln : Math  Operator=log  SaturateOnIntegerOverflow=on
  ln1 : Math  Operator=log  SaturateOnIntegerOverflow=on
  Out1 : Outport
  wires:
  Switch/1 -> Out1/1
  [Tmean] -> Add/1, Product/1
  Constant/1 -> Product/2
  Product/1 -> Divide/1
  Add/1 -> Divide/2
  Constant1/1 -> Add/2
  Divide/1 -> Subtract/3, Add1/1
  ln/1 -> Add1/2, Subtract/2
  Divide1/1 -> ln/1
  [RHmean] -> Divide1/1
  Constant2/1 -> Divide1/2
  Add1/1 -> Divide2/2
  Constant4/1 -> Divide2/1
  Constant3/1 -> Subtract/1
  Subtract/1 -> Divide2/3
  Divide2/1 -> Switch/1
  [Tmean] -> Add2/1, Product1/1
  Product1/1 -> Divide3/1
  Constant8/1 -> Subtract1/1
  [RHmean] -> Divide4/1
  Constant5/1 -> Product1/2
  Add2/1 -> Divide3/2
  Divide3/1 -> Subtract1/3, Add3/1
  ln1/1 -> Add3/2, Subtract1/2
  Constant6/1 -> Add2/2
  Subtract1/1 -> Divide5/3
  Divide4/1 -> ln1/1
  Constant7/1 -> Divide4/2
  [Tmean] -> Switch/2
  Constant9/1 -> Divide5/1
  Add3/1 -> Divide5/2
  Divide5/1 -> Switch/3

== system cop/COP/Climate Model/ Final Calculation for Data/Daily Temperature [°C]/Mean Air Temperature at 2m height (Tmean) [°C] ==
  In1 : Inport
  Out1 : Outport
  wires:
  In1/1 -> Out1/1

== system cop/COP/Climate Model/ Final Calculation for Data/Net Radiation at the Crop Surface (Rn) [MJ//m^2//day]/Clear-Sky Solar Radiation (Rso) [MJ//m^2//day] ==
  Add : Sum
  Constant : Constant  Value=0.75
  Constant1 : Constant  Value=0.00002
  Product : Product
  Product1 : Product
  Rso : Outport
  wires:
  Product/1 -> Rso/1
  [Ra] -> Product/2
  Add/1 -> Product/1
  Constant/1 -> Add/1
  Product1/1 -> Add/2
  [Altitude] -> Product1/2
  Constant1/1 -> Product1/1

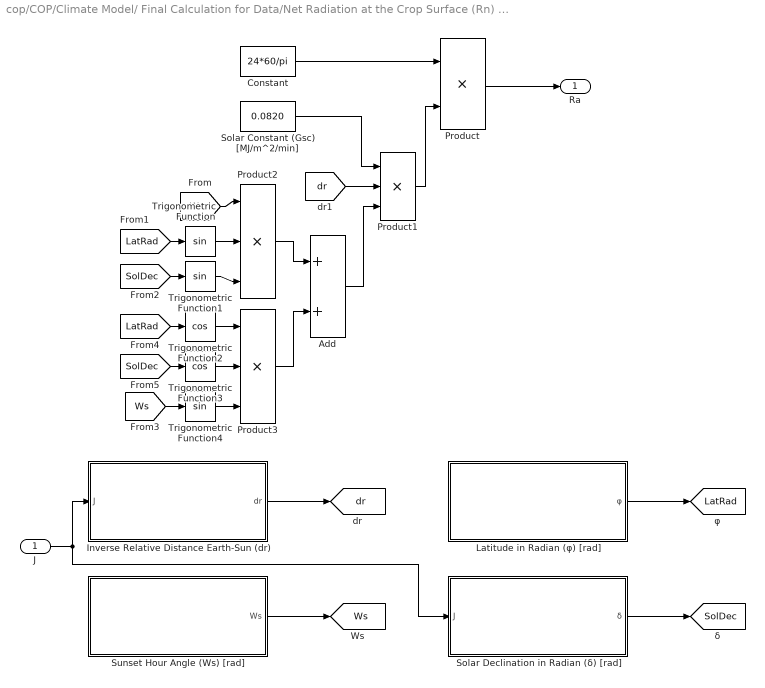
== system cop/COP/Climate Model/ Final Calculation for Data/Net Radiation at the Crop Surface (Rn) [MJ//m^2//day]/Extraterrestrial Radiation (Ra) [MJ//m^2//day] ==
  J : Inport
  Add : Sum
  Constant : Constant  Value=24*60/pi
  Inverse Relative Distance Earth-Sun (dr) : Subsystem
  Latitude in Radian (φ) [rad] : Subsystem
  Product : Product
  Product1 : Product  Inputs=3
  Product2 : Product  Inputs=3
  Product3 : Product  Inputs=3
  Solar Constant (Gsc) [MJ/m^2/min] : Constant  Value=0.0820
  Solar Declination in Radian (δ) [rad] : Subsystem
  Sunset Hour Angle (Ws) [rad] : Subsystem
  Trigonometric Function : Trigonometry
  Trigonometric Function1 : Trigonometry
  Trigonometric Function2 : Trigonometry  Operator=cos
  Trigonometric Function3 : Trigonometry  Operator=cos
  Trigonometric Function4 : Trigonometry
  Ra : Outport
  tag scope: LatRad=global, SolDec=global, Ws=global, dr=global
  wires:
  Constant/1 -> Product/1
  Product/1 -> Ra/1
  Product1/1 -> Product/2
  Solar Constant (Gsc) [MJ/m^2/min]/1 -> Product1/1
  Latitude in Radian (φ) [rad]/1(φ) -> [LatRad]
  Solar Declination in Radian (δ) [rad]/1(δ) -> [SolDec]
  Sunset Hour Angle (Ws) [rad]/1(Ws) -> [Ws]
  Inverse Relative Distance Earth-Sun (dr)/1(dr) -> [dr]
  [dr] -> Product1/2
  Trigonometric Function/1 -> Product2/2
  Trigonometric Function1/1 -> Product2/3
  [Ws] -> Product2/1
  [LatRad] -> Trigonometric Function/1
  [SolDec] -> Trigonometric Function1/1
  Product2/1 -> Add/1
  Add/1 -> Product1/3
  [SolDec] -> Trigonometric Function3/1
  [LatRad] -> Trigonometric Function2/1
  Product3/1 -> Add/2
  Trigonometric Function2/1 -> Product3/1
  Trigonometric Function3/1 -> Product3/2
  Trigonometric Function4/1 -> Product3/3
  [Ws] -> Trigonometric Function4/1
  J/1 -> Solar Declination in Radian (δ) [rad]/1(J), Inverse Relative Distance Earth-Sun (dr)/1(J)

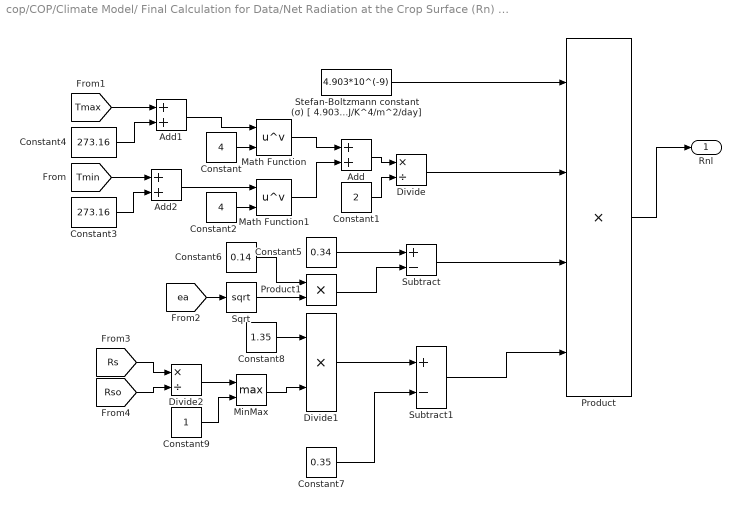
== system cop/COP/Climate Model/ Final Calculation for Data/Net Radiation at the Crop Surface (Rn) [MJ//m^2//day]/Net Longwave Radiation (Rnl) [MJ//m^2//day] ==
  Add : Sum
  Add1 : Sum
  Add2 : Sum
  Constant : Constant  Value=4
  Constant1 : Constant  Value=2
  Constant2 : Constant  Value=4
  Constant3 : Constant  Value=273.16
  Constant4 : Constant  Value=273.16
  Constant5 : Constant  Value=0.34
  Constant6 : Constant  Value=0.14
  Constant7 : Constant  Value=0.35
  Constant8 : Constant  Value=1.35
  Constant9 : Constant
  Divide : Product  Inputs=*/
  Divide1 : Product  Inputs=**
  Divide2 : Product  Inputs=*/
  Math Function : Math  Operator=pow  SaturateOnIntegerOverflow=on
  Math Function1 : Math  Operator=pow  SaturateOnIntegerOverflow=on
  MinMax : MinMax  Function=max  Inputs=2
  Product : Product  Inputs=4
  Product1 : Product
  Sqrt : Sqrt  SaturateOnIntegerOverflow=on
  Stefan-Boltzmann constant (σ) [ 4.903 10^-9 MJ/K^4/m^2/day] : Constant  Value=4.903*10^(-9)
  Subtract : Sum  Inputs=+-
  Subtract1 : Sum  Inputs=+-
  Rnl : Outport
  wires:
  Product/1 -> Rnl/1
  Stefan-Boltzmann constant (σ) [ 4.903 10^-9 MJ/K^4/m^2/day]/1 -> Product/1
  Constant/1 -> Math Function/2
  Math Function/1 -> Add/1
  Add/1 -> Divide/1
  Divide/1 -> Product/2
  Constant1/1 -> Divide/2
  Math Function1/1 -> Add/2
  Constant2/1 -> Math Function1/2
  Add1/1 -> Math Function/1
  Add2/1 -> Math Function1/1
  Constant3/1 -> Add2/2
  Constant4/1 -> Add1/2
  [Tmin] -> Add2/1
  [Tmax] -> Add1/1
  Subtract/1 -> Product/3
  Constant5/1 -> Subtract/1
  Product1/1 -> Subtract/2
  Constant6/1 -> Product1/1
  Sqrt/1 -> Product1/2
  [ea] -> Sqrt/1
  Subtract1/1 -> Product/4
  Divide1/1 -> Subtract1/1
  Constant7/1 -> Subtract1/2
  Constant8/1 -> Divide1/1
  [Rs] -> Divide2/1
  [Rso] -> Divide2/2
  Divide2/1 -> MinMax/1
  MinMax/1 -> Divide1/2
  Constant9/1 -> MinMax/2

== system cop/COP/Climate Model/ Final Calculation for Data/Net Radiation at the Crop Surface (Rn) [MJ//m^2//day]/Net Solar//Shortwave Radiation (Rns) [MJ//m^2//day] ==
  Albedo or canopy reflection coefficient for the reference crop (G) : Subsystem
  Constant : Constant
  Product : Product
  Subtract : Sum  Inputs=+-
  Out1 : Outport
  wires:
  Product/1 -> Out1/1
  Constant/1 -> Subtract/1
  Albedo or canopy reflection coefficient for the reference crop (G)/1(Out1) -> Subtract/2
  Subtract/1 -> Product/1
  [Rs] -> Product/2

== system cop/COP/Climate Model/ Final Calculation for Data/Net Radiation at the Crop Surface (Rn) [MJ//m^2//day]/Solar Radiation (Rs) [MJ//m^2//day] ==
  Actual Duration of Sunlight (n) [hour] : Constant  Value=12
  Angstrom Formula if AI_Rs not avaliable : Subsystem
  Constant : Constant  Value=Ac_Rs
  Hargreaves Formula if AI_Rs and hour of daylight is not available : Subsystem  mask{kRs=0.16}
      mask prompts: kRs "Adjustment Coefficient"
      mask DialogControl Control2 Prompt: The square root of the temperature difference is closely related to the existing daily solar radiation in a given location. The adjustment coefficient kRs is empirical and differs for 'interior' or 'coastal' regions:
      mask DialogControl Control3 Prompt: · for 'interior' locations, where land mass dominates and air masses are not strongly influenced by a large water body, kRs @ 0.16;
      mask DialogControl Control4 Prompt: · for 'coastal' locations, situated on or adjacent to the coast of a large land mass and where air masses are influenced by a nearby water body, kRs @ 0.19.
  Index Vector : MultiPortSwitch
  Rs : Outport
  wires:
  Constant/1 -> Index Vector/1
  [AI_Rs] -> Index Vector/2
  Angstrom Formula if AI_Rs not avaliable/1(Out1) -> Index Vector/3
  Index Vector/1 -> Rs/1
  Hargreaves Formula if AI_Rs and hour of daylight is not available/1(Rs) -> Index Vector/4
  Actual Duration of Sunlight (n) [hour]/1 -> Angstrom Formula if AI_Rs not avaliable/1(In1)
